simulink model "RocketBooster_P2"  (R2024b)
settings: Solver=VariableStepAuto  StartTime=0.0  StopTime=10.0  RelTol=1e-3
undefined symbols (not defined in the file): A, alpha0, B, C, Cd, D, Dd, dFT_test, H, Phi, Ts, x0
settings Model: Creator=maria  LastModifiedBy=maria

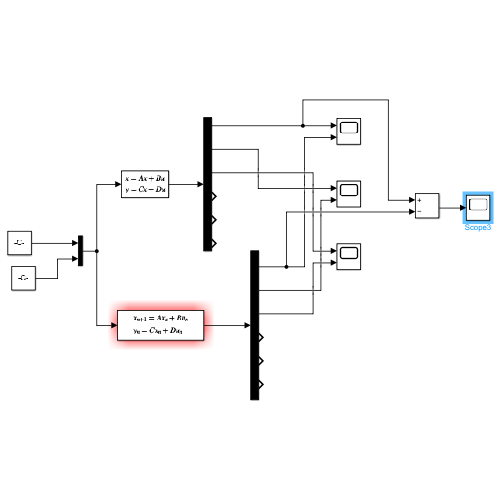
[thumbnail: Simulink's stored preview of the top-level diagram]
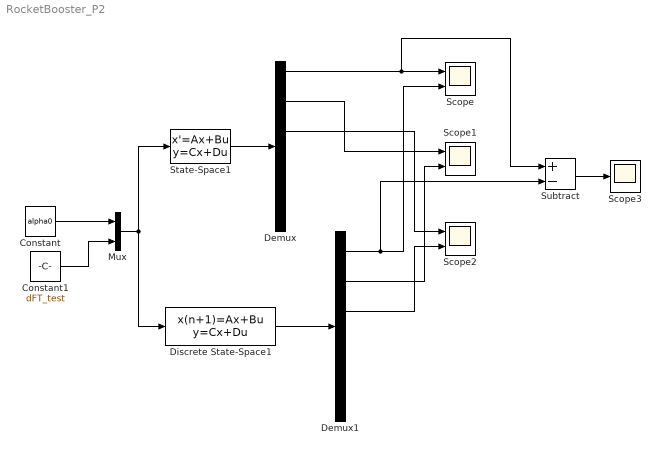
== system RocketBooster_P2 ==
  Constant : Constant  Value=alpha0
  Constant1 : Constant  Value=dFT_test
  Demux : Demux  Outputs=6
  Demux1 : Demux  Outputs=6
  Discrete State-Space1 : DiscreteStateSpace  A=Phi  B=H  C=Cd  D=Dd  InitialCondition=x0  SampleTime=Ts
  Mux : Mux  Inputs=2
  Scope : Scope  NumInputPorts=2
  Scope1 : Scope  NumInputPorts=2
  Scope2 : Scope  NumInputPorts=2
  Scope3 : Scope
  State-Space1 : StateSpace  A=A  B=B  C=C  D=D  InitialCondition=x0
  Subtract : Sum  Inputs=+-
  wires:
  Constant/1 -> Mux/1
  Mux/1 -> Discrete State-Space1/1, State-Space1/1
  Constant1/1 -> Mux/2
  State-Space1/1 -> Demux/1
  Discrete State-Space1/1 -> Demux1/1
  Demux1/1 -> Subtract/2, Scope/2
  Demux/1 -> Subtract/1, Scope/1
  Demux/2 -> Scope1/1
  Demux1/2 -> Scope1/2
  Demux/3 -> Scope2/1
  Demux1/3 -> Scope2/2
  Subtract/1 -> Scope3/1
